simulink model "s_2dsfl_pos_cntrl"  (R2021a)
settings: Solver=ode1  StartTime=0.0  StopTime=15  FixedStep=0.002  RelTol=1e-3  EnableMultiTasking=on
values from neighbouring files (symbols this model uses):
  A1 = [0 0 0 0 0 0 628.889014083 -863.33243061 1 0 -62.9562756075 62.9562756075 ... (16 elements, 4x4)]    [lqr_full_10deg.mat]
  A2 = [0 0 0 0 0 0 2271.11688578 -3336.19989408 1 0 -496.762762663 496.762762663 ... (16 elements, 4x4)]    [lqr_full_10deg.mat]
  B1 = [0 0 140.471189949 -140.471189949]    [lqr_full_10deg.mat]
  B2 = [0 0 288.122402345 -288.122402345]    [lqr_full_10deg.mat]
  C1 = [1 0 0 0 0 1 0 0 0 0 1 0 ... (16 elements, 4x4)]    [lqr_full_10deg.mat]
  C2 = [1 0 0 0 0 1 0 0 0 0 1 0 ... (16 elements, 4x4)]    [lqr_full_10deg.mat]
  D1 = [0 0 0 0]    [lqr_full_10deg.mat]
  D2 = [0 0 0 0]    [lqr_full_10deg.mat]
  K1 = [15.8113883008 -42.9312660346 2.18252832201 -0.706541352238]    [lqr_full_10deg.mat]
  K2 = [15.8113883008 -40.334902222 0.423884656834 -0.710902602847]    [lqr_full_10deg.mat]
undefined symbols (not defined in the file or in its folder): qc_get_step_size
libraries: simulink_extras x6, quarc_library x2
settings Model: ExtModeTrigDuration=5000  Creator=MLevis  LastModifiedBy=hurak
settings SolverCC: AlgebraicLoopSolver=TrustRegion  PositivePriorityOrder=on
settings DataIOCC: LimitDataPoints=on  SaveFormat=Array  SignalLoggingSaveFormat=ModelDataLogs  ReturnWorkspaceOutputs=off
settings OptimizationCC: ExpressionDepthLimit=2147483647  InitFltsAndDblsToZero=on
settings DebuggingCC: UnderspecifiedInitializationDetection=Classic  MergeDetectMultiDrivingBlocksExec=none  SolverPrmCheckMsg=warning  FcnCallInpInsideContextMsg=warning  StateNameClashWarn=warning  SFUnexpectedBacktrackingDiag=warning  SFNoUnconditionalDefaultTransitionDiag=warning  SFExecutionAtInitializationDiag=none  SFMachineParentedDataDiag=warning  ArithmeticOperatorsInVariantConditions=warning
settings HardwareCC: ProdBitPerPointer=32  ProdBitPerSizeT=32  ProdBitPerPtrDiffT=32  ProdWordSize=32  ProdHWDeviceType=Intel->x86-32 (Windows32)
settings ModelReferenceCC: PropagateSignalLabelsOutOfModel=off
settings RTWCC: Description=QUARC Win32 Target Using Toolchain  SystemTargetFile=quarc_windows.tlc  TemplateMakefile=quarc_default_tmf  Toolchain=QUARC windows | nmake (64-bit Windows)  BuildConfiguration=Faster Runs
settings CodeAppCC: StateflowObjectComments=on
settings STFCustomTargetCC: ConcurrentExecutionCompliant=on  SystemTargetFile=quarc_windows.tlc
settings GRTTargetCC: TargetLangStandard=C89/C90 (ANSI)  ParMdlRefBuildCompliant=off  CompOptLevelCompliant=off  CombineOutputUpdateFcns=off  MatFileLogging=off  CPPClassGenCompliant=off  GRTInterface=on  ExtMode=on  ExtModeMexFile=quarc_comm
settings ConfigComp: CovMetricSettings=dw  CovSaveCumulativeToWorkspaceVar=on  CovSaveSingleToWorkspaceVar=on

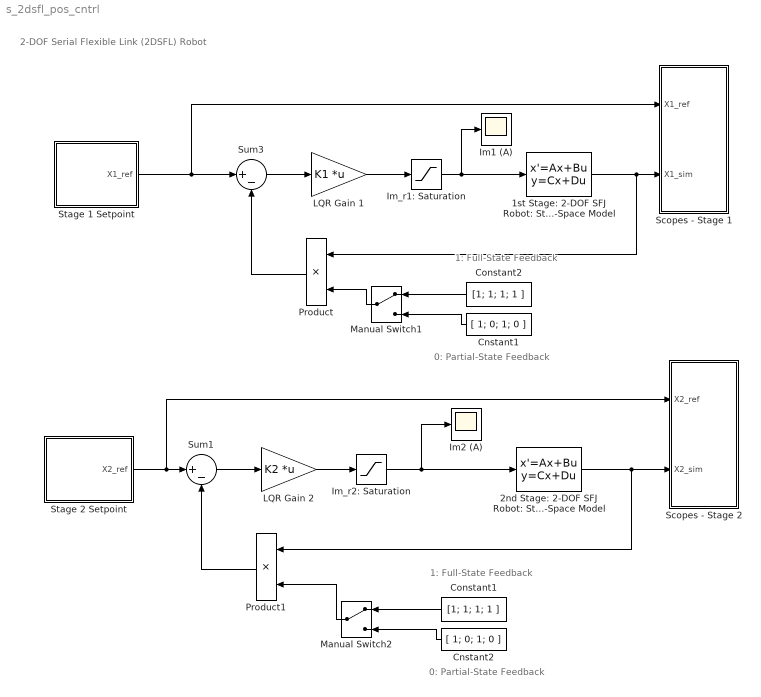
== system s_2dsfl_pos_cntrl ==
  note: 1: Full-State Feedback
  note: 0: Partial-State Feedback
  note: 1: Full-State Feedback
  note: 0: Partial-State Feedback
  note: 2-DOF Serial Flexible Link (2DSFL) Robot
  1st Stage: 2-DOF SFJ Robot: State-Space Model : StateSpace  A=A1  B=B1  C=C1  D=D1  InitialCondition=0
  2nd Stage: 2-DOF SFJ Robot: State-Space Model : StateSpace  A=A2  B=B2  C=C2  D=D2  InitialCondition=0
  Cnstant1 : Constant  Value=[ 1; 0; 1; 0 ]
  Cnstant2 : Constant  Value=[ 1; 0; 1; 0 ]
  Constant1 : Constant  Value=[1; 1; 1; 1 ]
  Constant2 : Constant  Value=[1; 1; 1; 1 ]
  Im1 (A) : Scope
  Im2 (A) : Scope
  Im_r1: Saturation : Saturate  UpperLimit=0.94  LowerLimit=-0.94
  Im_r2: Saturation : Saturate  UpperLimit=1.2  LowerLimit=-1.2
  LQR Gain 1 : Gain  Gain=K1  Multiplication=Matrix(K*u)
  LQR Gain 2 : Gain  Gain=K2  Multiplication=Matrix(K*u)
  Manual Switch1 : ManualSwitch
  Manual Switch2 : ManualSwitch
  Product : Product  InputSameDT=on  RndMeth=Zero  SaturateOnIntegerOverflow=on  OutDataTypeStr=Inherit: Same as first input
  Product1 : Product  InputSameDT=on  RndMeth=Zero  SaturateOnIntegerOverflow=on  OutDataTypeStr=Inherit: Same as first input
  Scopes - Stage 1 : Subsystem
  Scopes - Stage 2 : Subsystem
  Stage 1 Setpoint : Subsystem
  Stage 2 Setpoint : Subsystem
  Sum1 : Sum  Inputs=|+-  InputSameDT=on  SaturateOnIntegerOverflow=on  OutDataTypeStr=Inherit: Same as first input
  Sum3 : Sum  Inputs=|+-  InputSameDT=on  SaturateOnIntegerOverflow=on  OutDataTypeStr=Inherit: Same as first input
  wires:
  Constant2/1 -> Manual Switch1/1
  Cnstant1/1 -> Manual Switch1/2
  Manual Switch1/1 -> Product/2
  1st Stage: 2-DOF SFJ Robot: State-Space Model/1 -> Product/1, Scopes - Stage 1/2(X1_sim)
  Product/1 -> Sum3/2
  Stage 1 Setpoint/1(X1_ref) -> Sum3/1, Scopes - Stage 1/1(X1_ref)
  Sum3/1 -> LQR Gain 1/1
  LQR Gain 1/1 -> Im_r1: Saturation/1
  Im_r1: Saturation/1 -> 1st Stage: 2-DOF SFJ Robot: State-Space Model/1, Im1 (A)/1
  Product1/1 -> Sum1/2
  Sum1/1 -> LQR Gain 2/1
  Stage 2 Setpoint/1(X2_ref) -> Sum1/1, Scopes - Stage 2/1(X2_ref)
  LQR Gain 2/1 -> Im_r2: Saturation/1
  Im_r2: Saturation/1 -> 2nd Stage: 2-DOF SFJ Robot: State-Space Model/1, Im2 (A)/1
  2nd Stage: 2-DOF SFJ Robot: State-Space Model/1 -> Scopes - Stage 2/2(X2_sim), Product1/1
  Constant1/1 -> Manual Switch2/1
  Cnstant2/1 -> Manual Switch2/2
  Manual Switch2/1 -> Product1/2

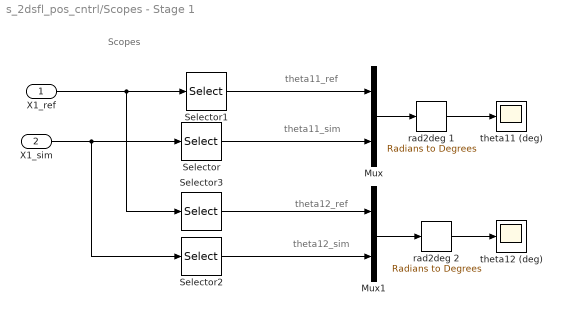
== system s_2dsfl_pos_cntrl/Scopes - Stage 1 ==
  note: theta11_sim
  note: theta11_ref
  note: theta12_sim
  note: Scopes
  note: theta12_ref
  X1_ref : Inport
  X1_sim : Inport  Port=2
  Mux : Mux  Inputs=2
  Mux1 : Mux  Inputs=2
  Selector : Selector  InputPortWidth=4  IndexOptions=Index vector (dialog)  Indices=[1]  OutputSizes=1
  Selector1 : Selector  InputPortWidth=4  IndexOptions=Index vector (dialog)  Indices=[1]  OutputSizes=1
  Selector2 : Selector  InputPortWidth=4  IndexOptions=Index vector (dialog)  Indices=[2]  OutputSizes=1
  Selector3 : Selector  InputPortWidth=4  IndexOptions=Index vector (dialog)  Indices=[2]  OutputSizes=1
  rad2deg 1 : simulink_extras/Transformations/Radians to Degrees  SystemSampleTime=-1
  rad2deg 2 : simulink_extras/Transformations/Radians to Degrees  SystemSampleTime=-1
  theta11 (deg) : Scope
  theta12 (deg) : Scope
  wires:
  Selector2/1 -> Mux1/2
  Selector/1 -> Mux/2
  rad2deg 2/1 -> theta12 (deg)/1
  rad2deg 1/1 -> theta11 (deg)/1
  X1_sim/1 -> Selector2/1, Selector/1
  Mux/1 -> rad2deg 1/1
  X1_ref/1 -> Selector1/1, Selector3/1
  Mux1/1 -> rad2deg 2/1
  Selector1/1 -> Mux/1
  Selector3/1 -> Mux1/1

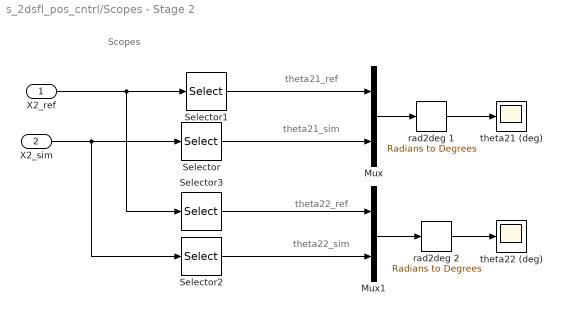
== system s_2dsfl_pos_cntrl/Scopes - Stage 2 ==
  note: theta22_ref
  note: Scopes
  note: theta22_sim
  note: theta21_ref
  note: theta21_sim
  X2_ref : Inport
  X2_sim : Inport  Port=2
  Mux : Mux  Inputs=2
  Mux1 : Mux  Inputs=2
  Selector : Selector  InputPortWidth=4  IndexOptions=Index vector (dialog)  Indices=[1]  OutputSizes=1
  Selector1 : Selector  InputPortWidth=4  IndexOptions=Index vector (dialog)  Indices=[1]  OutputSizes=1
  Selector2 : Selector  InputPortWidth=4  IndexOptions=Index vector (dialog)  Indices=[2]  OutputSizes=1
  Selector3 : Selector  InputPortWidth=4  IndexOptions=Index vector (dialog)  Indices=[2]  OutputSizes=1
  rad2deg 1 : simulink_extras/Transformations/Radians to Degrees  SystemSampleTime=-1
  rad2deg 2 : simulink_extras/Transformations/Radians to Degrees  SystemSampleTime=-1
  theta21 (deg) : Scope
  theta22 (deg) : Scope
  wires:
  Selector3/1 -> Mux1/1
  Selector1/1 -> Mux/1
  Mux1/1 -> rad2deg 2/1
  X2_ref/1 -> Selector3/1, Selector1/1
  Mux/1 -> rad2deg 1/1
  X2_sim/1 -> Selector/1, Selector2/1
  rad2deg 1/1 -> theta21 (deg)/1
  rad2deg 2/1 -> theta22 (deg)/1
  Selector/1 -> Mux/2
  Selector2/1 -> Mux1/2

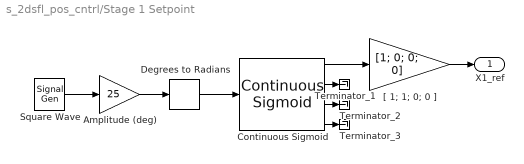
== system s_2dsfl_pos_cntrl/Stage 1 Setpoint ==
  Amplitude (deg) : Gain  Gain=25  SaturateOnIntegerOverflow=on  OutDataTypeStr=Inherit: Same as input  ParamDataTypeStr=Inherit: Same as input
  Continuous Sigmoid : quarc_library/Sources/Sigmoids/Continuous Sigmoid  params_source=Internal (dialog parameters)  max_velocity=2.35  max_acceleration=4.45  initial_position=0  initial_velocity=0  hold_off=0.5  input_sample_time=-1  output_sample_time=qc_get_step_size
      settings: SourceProductName=QUARC Targets
  Degrees to Radians : simulink_extras/Transformations/Degrees to Radians  SystemSampleTime=-1
  Square Wave : SignalGenerator  WaveForm=square  Frequency=0.1
  Terminator_1 : Terminator
  Terminator_2 : Terminator
  Terminator_3 : Terminator
  "[ 1; 1; 0; 0 ]" : Gain  Gain=[1; 0; 0; 0]  SaturateOnIntegerOverflow=on  OutDataTypeStr=Inherit: Same as input  ParamDataTypeStr=Inherit: Same as input
  X1_ref : Outport
  wires:
  Square Wave/1 -> Amplitude (deg)/1
  Amplitude (deg)/1 -> Degrees to Radians/1
  "[ 1; 1; 0; 0 ]"/1 -> X1_ref/1
  Degrees to Radians/1 -> Continuous Sigmoid/1
  Continuous Sigmoid/2 -> Terminator_1/1
  Continuous Sigmoid/3 -> Terminator_2/1
  Continuous Sigmoid/4 -> Terminator_3/1
  Continuous Sigmoid/1 -> "[ 1; 1; 0; 0 ]"/1

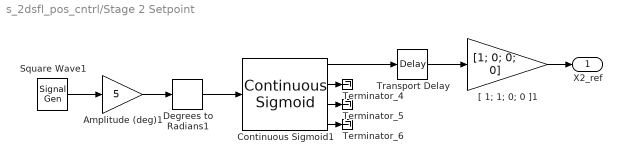
== system s_2dsfl_pos_cntrl/Stage 2 Setpoint ==
  Amplitude (deg)1 : Gain  Gain=5  SaturateOnIntegerOverflow=on  OutDataTypeStr=Inherit: Same as input  ParamDataTypeStr=Inherit: Same as input
  Continuous Sigmoid1 : quarc_library/Sources/Sigmoids/Continuous Sigmoid  params_source=Internal (dialog parameters)  max_velocity=2  max_acceleration=5  initial_position=0  initial_velocity=0  hold_off=0.5  input_sample_time=-1  output_sample_time=qc_get_step_size
      settings: SourceProductName=QUARC Targets
  Degrees to Radians1 : simulink_extras/Transformations/Degrees to Radians  SystemSampleTime=-1
  Square Wave1 : SignalGenerator  WaveForm=square  Frequency=0.1
  Terminator_4 : Terminator
  Terminator_5 : Terminator
  Terminator_6 : Terminator
  Transport Delay : TransportDelay  DelayTime=2.5  BufferSize=10/qc_get_step_size
  "[ 1; 1; 0; 0 ]1" : Gain  Gain=[1; 0; 0; 0]  SaturateOnIntegerOverflow=on  OutDataTypeStr=Inherit: Same as input  ParamDataTypeStr=Inherit: Same as input
  X2_ref : Outport
  wires:
  Continuous Sigmoid1/1 -> Transport Delay/1
  Transport Delay/1 -> "[ 1; 1; 0; 0 ]1"/1
  Square Wave1/1 -> Amplitude (deg)1/1
  Amplitude (deg)1/1 -> Degrees to Radians1/1
  Continuous Sigmoid1/2 -> Terminator_4/1
  Continuous Sigmoid1/3 -> Terminator_5/1
  Continuous Sigmoid1/4 -> Terminator_6/1
  Degrees to Radians1/1 -> Continuous Sigmoid1/1
  "[ 1; 1; 0; 0 ]1"/1 -> X2_ref/1
